simulink model "CBF_Attitude_with_feedback"  (R2020b)
settings: Solver=ode113  StartTime=0.0  StopTime=4  RelTol=1e-3
settings Model: Creator=kt012  LastModifiedBy=kt012

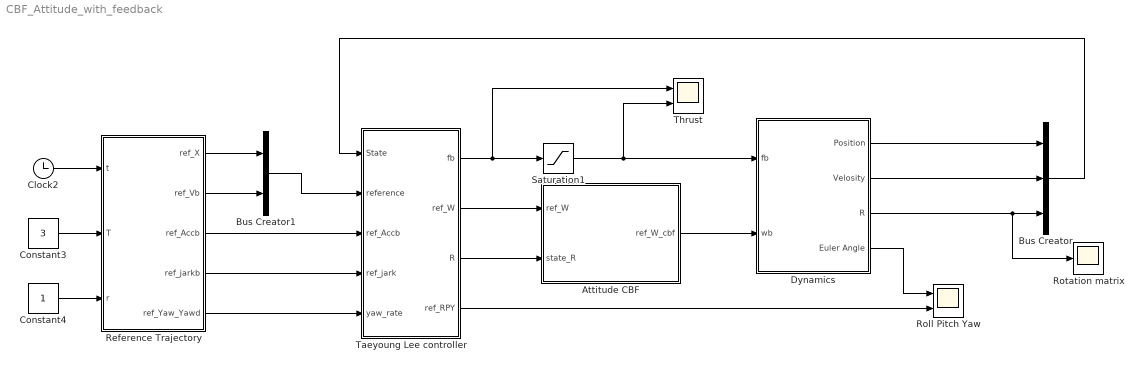
== system CBF_Attitude_with_feedback ==
  Attitude CBF : Subsystem
  Bus Creator : BusCreator  Inputs=3
  Bus Creator1 : BusCreator  Inputs=2
  Clock2 : Clock
  Constant3 : Constant  Value=3
  Constant4 : Constant
  Dynamics : Subsystem
  Reference Trajectory : MATLAB Function  TreatAsAtomicUnit=on
  Roll Pitch Yaw : Scope  NumInputPorts=2
  Rotation matrix : Scope
  Saturation1 : Saturate  UpperLimit=9.8*1.5
  Taeyoung Lee controller : Subsystem
  Thrust : Scope  NumInputPorts=2
  wires:
  Dynamics/2(Velosity) -> Bus Creator/2
  Taeyoung Lee controller/1(fb) -> Saturation1/1, Thrust/1
  Constant3/1 -> Reference Trajectory/2(T)
  Constant4/1 -> Reference Trajectory/3(r)
  Dynamics/4(Euler Angle) -> Roll Pitch Yaw/1
  Taeyoung Lee controller/2(ref_W) -> Attitude CBF/1(ref_W)
  Reference Trajectory/4(ref_jarkb) -> Taeyoung Lee controller/4(ref_jark)
  Reference Trajectory/1(ref_X) -> Bus Creator1/1
  Bus Creator/1 -> Taeyoung Lee controller/1(State)
  Reference Trajectory/2(ref_Vb) -> Bus Creator1/2
  Reference Trajectory/5(ref_Yaw_Yawd) -> Taeyoung Lee controller/5(yaw_rate)
  Dynamics/3(R) -> Rotation matrix/1, Bus Creator/3
  Reference Trajectory/3(ref_Accb) -> Taeyoung Lee controller/3(ref_Accb)
  Saturation1/1 -> Thrust/2, Dynamics/1(fb)
  Clock2/1 -> Reference Trajectory/1(t)
  Dynamics/1(Position) -> Bus Creator/1
  Bus Creator1/1 -> Taeyoung Lee controller/2(reference)
  Taeyoung Lee controller/4(ref_RPY) -> Roll Pitch Yaw/2
  Attitude CBF/1(ref_W_cbf) -> Dynamics/2(wb)
  Taeyoung Lee controller/3(R) -> Attitude CBF/2(state_R)

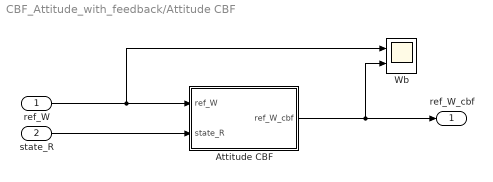
== system CBF_Attitude_with_feedback/Attitude CBF ==
  ref_W : Inport
  state_R : Inport  Port=2
  Attitude CBF : MATLAB Function  TreatAsAtomicUnit=on
  Wb : Scope  NumInputPorts=2
  ref_W_cbf : Outport
  wires:
  state_R/1 -> Attitude CBF/2(state_R)
  ref_W/1 -> Attitude CBF/1(ref_W), Wb/1
  Attitude CBF/1(ref_W_cbf) -> ref_W_cbf/1, Wb/2

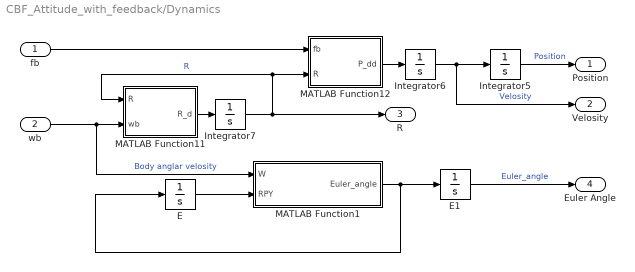
== system CBF_Attitude_with_feedback/Dynamics ==
  fb : Inport
  wb : Inport  Port=2
  E : Integrator  InitialCondition=[0 0 0];
  E1 : Integrator  InitialCondition=[0 0 0];
  Integrator5 : Integrator  InitialCondition=[0;0;0]
  Integrator6 : Integrator  InitialCondition=[0;0;0]
  Integrator7 : Integrator  InitialCondition=[1 0 0; 0 1 0; 0 0 1]
  MATLAB Function1 : MATLAB Function  TreatAsAtomicUnit=on
  MATLAB Function11 : MATLAB Function  TreatAsAtomicUnit=on
  MATLAB Function12 : MATLAB Function  TreatAsAtomicUnit=on
  Position : Outport
  Velosity : Outport  Port=2
  R : Outport  Port=3
  Euler Angle : Outport  Port=4
  wires:
  Integrator7/1 -> R/1, MATLAB Function12/2(R), MATLAB Function11/1(R)  "R"
  MATLAB Function11/1(R_d) -> Integrator7/1
  Integrator6/1 -> Velosity/1, Integrator5/1  "Velosity"
  MATLAB Function12/1(P_dd) -> Integrator6/1
  fb/1 -> MATLAB Function12/1(fb)
  Integrator5/1 -> Position/1  "Position"
  E/1 -> MATLAB Function1/2(RPY)
  E1/1 -> Euler Angle/1  "Euler_angle"
  MATLAB Function1/1(Euler_angle) -> E/1, E1/1
  wb/1 -> MATLAB Function1/1(W), MATLAB Function11/2(wb)  "Body anglar velosity"

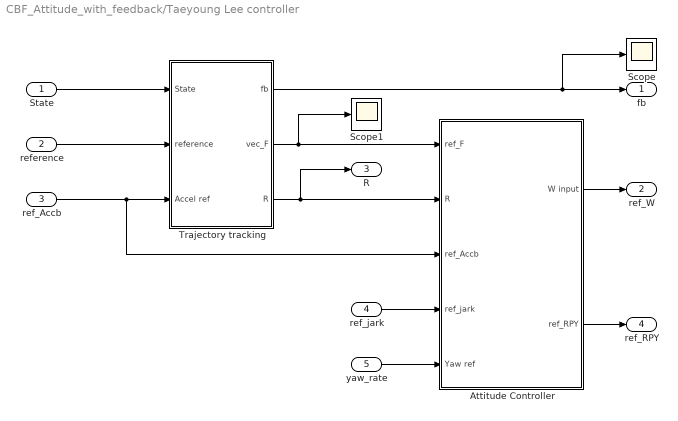
== system CBF_Attitude_with_feedback/Taeyoung Lee controller ==
  State : Inport
  reference : Inport  Port=2
  ref_Accb : Inport  Port=3
  ref_jark : Inport  Port=4
  yaw_rate : Inport  Port=5
  Attitude Controller : Subsystem
  Scope : Scope
  Scope1 : Scope
  Trajectory tracking : Subsystem
  fb : Outport
  ref_W : Outport  Port=2
  R : Outport  Port=3
  ref_RPY : Outport  Port=4
  wires:
  ref_Accb/1 -> Attitude Controller/3(ref_Accb), Trajectory tracking/3(Accel ref)
  ref_jark/1 -> Attitude Controller/4(ref_jark)
  reference/1 -> Trajectory tracking/2(reference)
  State/1 -> Trajectory tracking/1(State)
  yaw_rate/1 -> Attitude Controller/5(Yaw ref)
  Trajectory tracking/1(fb) -> Scope/1, fb/1
  Attitude Controller/1(W input) -> ref_W/1
  Trajectory tracking/2(vec_F) -> Scope1/1, Attitude Controller/1(ref_F)
  Attitude Controller/2(ref_RPY) -> ref_RPY/1
  Trajectory tracking/3(R) -> R/1, Attitude Controller/2(R)

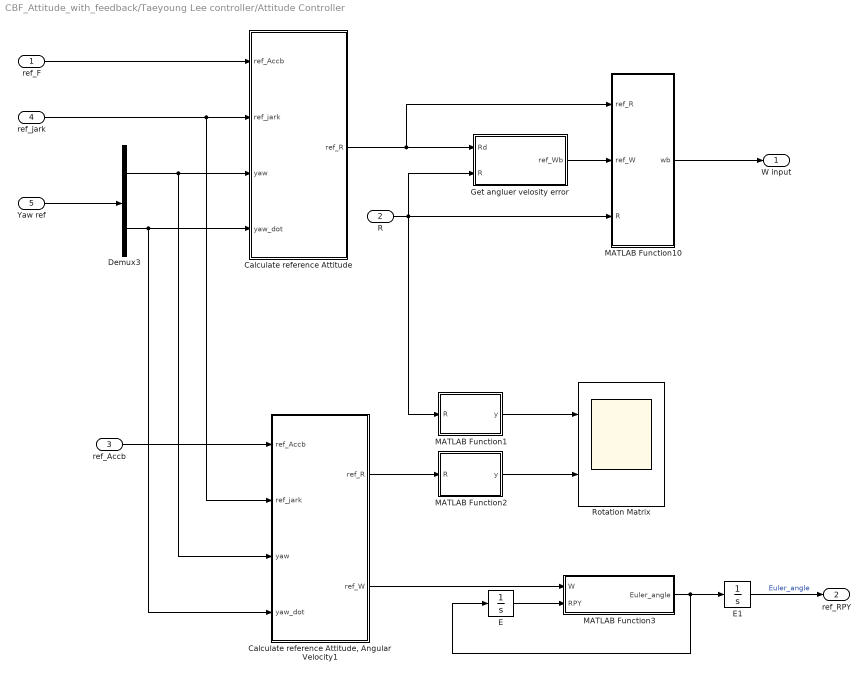
== system CBF_Attitude_with_feedback/Taeyoung Lee controller/Attitude Controller ==
  ref_F : Inport
  R : Inport  Port=2
  ref_Accb : Inport  Port=3
  ref_jark : Inport  Port=4
  Yaw ref : Inport  Port=5
  Calculate reference Attitude : MATLAB Function  TreatAsAtomicUnit=on
  "Calculate reference Attitude, Angular Velocity1" : MATLAB Function  TreatAsAtomicUnit=on
  Demux3 : Demux  Outputs=2
  E : Integrator  InitialCondition=[0 0 0];
  E1 : Integrator  InitialCondition=[0 0 0];
  Get angluer velosity error : Subsystem
  MATLAB Function1 : MATLAB Function  TreatAsAtomicUnit=on
  MATLAB Function10 : MATLAB Function  TreatAsAtomicUnit=on
  MATLAB Function2 : MATLAB Function  TreatAsAtomicUnit=on
  MATLAB Function3 : MATLAB Function  TreatAsAtomicUnit=on
  Rotation Matrix : Scope  NumInputPorts=2
  W input : Outport
  ref_RPY : Outport  Port=2
  wires:
  Demux3/2 -> Calculate reference Attitude/4(yaw_dot), "Calculate reference Attitude, Angular Velocity1"/4(yaw_dot)
  Yaw ref/1 -> Demux3/1
  Demux3/1 -> Calculate reference Attitude/3(yaw), "Calculate reference Attitude, Angular Velocity1"/3(yaw)
  ref_F/1 -> Calculate reference Attitude/1(ref_Accb)
  ref_jark/1 -> Calculate reference Attitude/2(ref_jark), "Calculate reference Attitude, Angular Velocity1"/2(ref_jark)
  MATLAB Function10/1(wb) -> W input/1
  MATLAB Function1/1(y) -> Rotation Matrix/1
  MATLAB Function2/1(y) -> Rotation Matrix/2
  ref_Accb/1 -> "Calculate reference Attitude, Angular Velocity1"/1(ref_Accb)
  "Calculate reference Attitude, Angular Velocity1"/1(ref_R) -> MATLAB Function2/1(R)
  "Calculate reference Attitude, Angular Velocity1"/2(ref_W) -> MATLAB Function3/1(W)
  MATLAB Function3/1(Euler_angle) -> E/1, E1/1
  E/1 -> MATLAB Function3/2(RPY)
  E1/1 -> ref_RPY/1  "Euler_angle"
  Calculate reference Attitude/1(ref_R) -> MATLAB Function10/1(ref_R), Get angluer velosity error/1(Rd)
  R/1 -> Get angluer velosity error/2(R), MATLAB Function10/3(R), MATLAB Function1/1(R)
  Get angluer velosity error/1(ref_Wb) -> MATLAB Function10/2(ref_W)

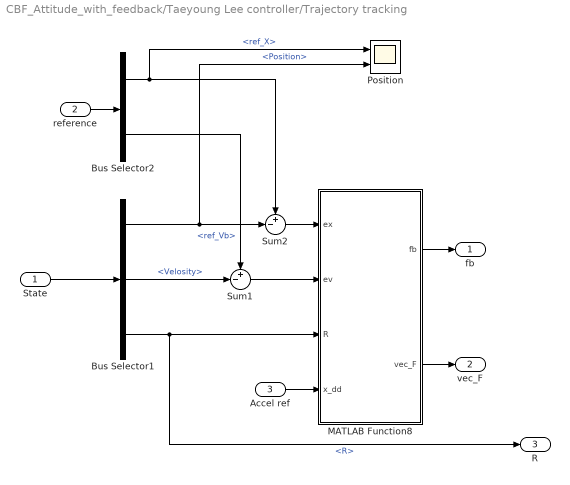
== system CBF_Attitude_with_feedback/Taeyoung Lee controller/Trajectory tracking ==
  State : Inport
  reference : Inport  Port=2
  Accel ref : Inport  Port=3
  Bus Selector1 : BusSelector  OutputSignals=Position,Velosity,R
  Bus Selector2 : BusSelector  OutputSignals=ref_X,ref_Vb
  MATLAB Function8 : MATLAB Function
  Position : Scope  NumInputPorts=2
  Sum1 : Sum  Inputs=+-|
  Sum2 : Sum  Inputs=+-|
  fb : Outport
  vec_F : Outport  Port=2
  R : Outport  Port=3
  wires:
  State/1 -> Bus Selector1/1
  Accel ref/1 -> MATLAB Function8/4(x_dd)
  reference/1 -> Bus Selector2/1
  MATLAB Function8/1(fb) -> fb/1
  MATLAB Function8/2(vec_F) -> vec_F/1
  Bus Selector2/2 -> Sum1/1  "<ref_Vb>"
  Bus Selector1/2 -> Sum1/2  "<Velosity>"
  Bus Selector2/1 -> Position/1, Sum2/1  "<ref_X>"
  Bus Selector1/1 -> Position/2, Sum2/2  "<Position>"
  Sum2/1 -> MATLAB Function8/1(ex)
  Bus Selector1/3 -> R/1, MATLAB Function8/3(R)  "<R>"
  Sum1/1 -> MATLAB Function8/2(ev)

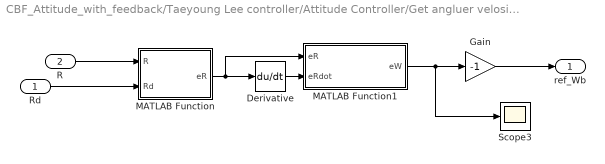
== system CBF_Attitude_with_feedback/Taeyoung Lee controller/Attitude Controller/Get angluer velosity error ==
  Rd : Inport
  R : Inport  Port=2
  Derivative : Derivative
  Gain : Gain  Gain=-1
  MATLAB Function : MATLAB Function  TreatAsAtomicUnit=on
  MATLAB Function1 : MATLAB Function  TreatAsAtomicUnit=on
  Scope3 : Scope
  ref_Wb : Outport
  wires:
  R/1 -> MATLAB Function/1(R)
  MATLAB Function/1(eR) -> MATLAB Function1/1(eR), Derivative/1
  MATLAB Function1/1(eW) -> Scope3/1, Gain/1
  Gain/1 -> ref_Wb/1
  Derivative/1 -> MATLAB Function1/2(eRdot)
  Rd/1 -> MATLAB Function/2(Rd)

== matlab function CBF_Attitude_with_feedback/Taeyoung Lee controller/Trajectory tracking/MATLAB Function8 ==
  data: ex input; fb output; ev input; R input; x_dd input; vec_F output
function [fb, vec_F]= fcn(ex,ev,R, x_dd)
ev_d = [0 0 0]';
ex_d = [0 0 0]';
fb = 0;
vec_F = [0 0 0]';
m = 1.0;
e3 = [0;0;1];

kx_x = 10;
kx_y = 10;
kx_z = 10;

kv_x = 10;
kv_y = 10;
kv_z = 10;

ex_x = kx_x*ex(1);
ex_y = kx_y*ex(2);
ex_z = kx_z*ex(3);
ex_d = [ex_x; ex_y; ex_z];

ev_x = kv_x*ev(1);
ev_y = kv_y*ev(2);
ev_z = kv_z*ev(3);
ev_d = [ev_x; ev_y; ev_z];
fb = dot(ex_d + ev_d + m*x_dd, R*e3);
tmp = ex_d + ev_d + m*x_dd;
if tmp(3) <= 0.0001
    tmp(3) = 0.0001;
end
vec_F = tmp;

== matlab function CBF_Attitude_with_feedback/Taeyoung Lee controller/Attitude Controller/MATLAB Function10 ==
  data: ref_R input; ref_W input; R input; wb output
function wb = fcn(ref_R,ref_W, R)
R_T = R';
Rd_T = ref_R';
eR = (Rd_T*R - R_T*ref_R)/2;

kR = 20;
wx = ref_W(1);
wy = ref_W(2);
wz = ref_W(3);
wd = [0 -wz wy; 
      wz 0 -wx;
      -wy wx 0];
u = -kR * eR + wd;

wb = u;

== matlab function CBF_Attitude_with_feedback/Dynamics/MATLAB Function12 ==
  data: fb input; P_dd output; R input
function P_dd = fcn(fb,R)
e3 = [0;0;1];
g = 9.8;
m = 1;

u = (fb*R*e3/m) - g*e3 ;

P_dd = u;

== matlab function CBF_Attitude_with_feedback/Reference Trajectory ==
  data: ref_X output; ref_Vb output; ref_Accb output; ref_jarkb output; t input; ref_Yaw_Yawd output; T input; r input
  function [ref_X, ref_Vb, ref_Accb, ref_jarkb, ref_Yaw_Yawd] = fcn(t,T,r)
% 軌道生成
w = 2 * pi/T;     
% 軌道生成（直線移動）
ref_X = [r*sin(w*t);0; 0];
ref_Vb = [r*w*cos(w*t); 0; 0];
ref_Accb = [-r*w^2*sin(w*t); 0; 9.8];
ref_jarkb = [-r*w^3*cos(w*t);0;0];
ref_Yaw_Yawd = [0, 0]'; 

% % 軌道生成（直線移動）
% ref_X = [r/(1+exp(-t));0; 0];
% ref_Vb = [(1-ref_X(1))*ref_X(1); 0; 0];
% ref_Accb = [(1-ref_Vb(1))*ref_Vb(1); 0; 9.8];
% ref_jarkb = [(1-ref_Accb(1))*ref_Accb(1);0;0];
% ref_Yaw_Yawd = [0, 0]';
% % 軌道生成
w = 2 * pi/T;     
% % 軌道生成（直線移動）
% ref_X = [1;0; 0];
% ref_Vb = [0; 0; 0];
% ref_Accb = [0; 0; 9.8];
% ref_jarkb = [-r*w^3*cos(w*t);0;0];
% ref_Yaw_Yawd = [0, 0]'; 

% 軌道生成（直線移動）
% ref_X = [4*t^2;0; 0];
% ref_Vb = [8*t; 0; 0];
% ref_Accb = [8; 0; 9.8];
% ref_jarkb = [0;0;0];
% ref_Yaw_Yawd = [0, 0]';

== matlab function CBF_Attitude_with_feedback/Taeyoung Lee controller/Attitude Controller/Calculate reference Attitude ==
  data: ref_R output; ref_Accb input; ref_jark input; yaw input; yaw_dot input
function ref_R= fcn(ref_Accb, ref_jark, yaw, yaw_dot)

% Flat Outputから内部状態と入力揚力を計算


Xc = [cos(yaw) sin(yaw) 0]';          % よー角のベクトル　Rc(3)
Yc = [-sin(yaw) cos(yaw) 0]';
dXc = yaw_dot * Yc; % よー角のベクトルの微分
dYc = -yaw_dot * Xc; 

% 所望の姿勢を計算している
% 軌道の加速度のベクトル: b3 を計算
Zb = ref_Accb / norm(ref_Accb);    
%
Yb = cross(Zb, Xc)/norm(cross(Zb, Xc));
Xb = cross(Yb, Zb);
% Xb = cross(Yc, Zb)/norm(cross(Yc, Zb));
% Yb = cross(Zb, Xb);
ref_R = [Xb Yb Zb] ;




% % 加加速度ベクトルを計算
% dfZb = ref_jark;
%   
% % 目標の姿勢のz軸方向のベクトルの微分を計算
% dZb = dfZb/norm(ref_Accb) - ref_Accb * dot(ref_Accb, dfZb)/norm(ref_Accb)^3; % Zb_dot---------- dot(　fb1/norm(fb1) )
% 
% % 目標の姿勢のx軸方向のベクトルを計算
% dnorm_Zb_Xc2 = norm(cross(dYc, Zb) + cross(Yc, dZb));
% dXb = (cross(dYc, Zb) + cross(Yc, dZb))/dnorm_Zb_Xc2 - cross(Yc, Zb) * dot(cross(Yc, Zb),( cross(dYc, Zb) + cross(Yc, dZb)))/dnorm_Zb_Xc2^3;
%    
% % 目標の姿勢のy軸方向のベクトルを計算
% dYb = cross(dZb, Xb) + cross(Zb, dXb) ;  %dot_b2 = dotb3とb1 の外積と　b3とdot_b1の外積　の和　--------- dot(cross(b3, b1))
% 
% 
% wy = dot(Xb, ref_jark) / dot(Zb, ref_Accb);
% wx = - dot(Yb, ref_jark) / dot(Zb, ref_Accb);
% wz = (yaw_dot * dot(Xc, Xb) + wy * dot(Yc, Zb))/norm(cross(Yc, Zb));
% ref_W = [wx wy wz];

== matlab function CBF_Attitude_with_feedback/Attitude CBF/Attitude CBF ==
  data: ref_W input; state_R input; ref_W_cbf output
function ref_W_cbf = fcn(ref_W, state_R)
ref_W = [ref_W(3, 2), -ref_W(3, 1), ref_W(2, 1)]';
theta = 0.5;
coder.extrinsic('quadprog')
tmp = zeros(3, 1);
e3 = [0; 0; 1];
e3_wedge = [0 -1 0; 1 0 0; 0 0 0];
H = eye(3);
f = -ref_W;
% ref_W
A = e3'*state_R*e3_wedge;
B = 10*(e3'*state_R*e3 - cos(theta));

tmp  = quadprog(H, f, A, B);
ref_W_cbf = [0      -tmp(3)   tmp(2); 
             tmp(3)  0       -tmp(1); 
             -tmp(2) tmp(1)   0]
A*tmp
B
end

== matlab function CBF_Attitude_with_feedback/Dynamics/MATLAB Function11 ==
  data: R input; wb input; R_d output
function R_d = fcn(R,wb)
u = R * wb;
R_d = u;

== matlab function CBF_Attitude_with_feedback/Taeyoung Lee controller/Attitude Controller/MATLAB Function2 ==
  data: R input; y output
function y = fcn(R)
Rtranspose = R';
eR = (R - Rtranspose)/2;

y = [eR(3, 2) -eR(3, 1) eR(2, 1)]';

== matlab function CBF_Attitude_with_feedback/Taeyoung Lee controller/Attitude Controller/MATLAB Function1 ==
  data: R input; y output
function y = fcn(R)
Rtranspose = R';
eR = (R - Rtranspose)/2;

y = [eR(3, 2) -eR(3, 1) eR(2, 1)]';

== matlab function CBF_Attitude_with_feedback/Taeyoung Lee controller/Attitude Controller/Calculate reference Attitude, Angular Velocity1 ==
  data: ref_R output; ref_W output; ref_Accb input; ref_jark input; yaw input; yaw_dot input
function [ref_R,ref_W]= fcn(ref_Accb, ref_jark, yaw, yaw_dot)

% Flat Outputから内部状態と入力揚力を計算


Xc = [cos(yaw) sin(yaw) 0]';          % よー角のベクトル　Rc(3)
Yc = [-sin(yaw) cos(yaw) 0]';
dXc = yaw_dot * Yc; % よー角のベクトルの微分
dYc = -yaw_dot * Xc; 

% 所望の姿勢を計算している
% 軌道の加速度のベクトル: b3 を計算
Zb = ref_Accb / norm(ref_Accb);   
%
Yb = cross(Zb, Xc)/norm(cross(Zb, Xc));
Xb = cross(Yb, Zb);
% Xb = cross(Yc, Zb)/norm(cross(Yc, Zb));
% Yb = cross(Zb, Xb);
ref_R = [Xb Yb Zb] ;
% 加加速度ベクトルを計算
dfZb = ref_jark;
  
% 目標の姿勢のz軸方向のベクトルの微分を計算
dZb = dfZb/norm(ref_Accb) - ref_Accb * dot(ref_Accb, dfZb)/norm(ref_Accb)^3; % Zb_dot---------- dot(　fb1/norm(fb1) )

% 目標の姿勢のx軸方向のベクトルを計算
dnorm_Zb_Xc2 = norm(cross(dYc, Zb) + cross(Yc, dZb));
dXb = (cross(dYc, Zb) + cross(Yc, dZb))/dnorm_Zb_Xc2 - cross(Yc, Zb) * dot(cross(Yc, Zb),( cross(dYc, Zb) + cross(Yc, dZb)))/dnorm_Zb_Xc2^3;
   
% 目標の姿勢のy軸方向のベクトルを計算
dYb = cross(dZb, Xb) + cross(Zb, dXb) ;  %dot_b2 = dotb3とb1 の外積と　b3とdot_b1の外積　の和　--------- dot(cross(b3, b1))


wy = dot(Xb, ref_jark) / dot(Zb, ref_Accb);
wx = - dot(Yb, ref_jark) / dot(Zb, ref_Accb);
wz = (yaw_dot * dot(Xc, Xb) + wy * dot(Yc, Zb))/norm(cross(Yc, Zb));
ref_W = [wx wy wz];

== matlab function CBF_Attitude_with_feedback/Taeyoung Lee controller/Attitude Controller/MATLAB Function3 ==
  data: W input; Euler_angle output; RPY input
function Euler_angle = fcn(W, RPY)
roll = RPY(1);
pitch = RPY(2);
yaw = RPY(3);
rollS = sin(roll); rollC = cos(roll);           
pitchS = sin(pitch); pitchC = cos(pitch);       


Euler_angle = pinv([1 0 -pitchS;
     0 rollC  pitchC * rollS;
     0 -rollS pitchC * rollC]) * W';

== matlab function CBF_Attitude_with_feedback/Dynamics/MATLAB Function1 ==
  data: W input; Euler_angle output; RPY input
function Euler_angle = fcn(W, RPY)
W = [W(3, 2), -W(3, 1), W(2, 1)]';
roll = RPY(1);
pitch = RPY(2);
yaw = RPY(3);
rollS = sin(roll); rollC = cos(roll);           
pitchS = sin(pitch); pitchC = cos(pitch);       


Euler_angle = pinv([1 0 -pitchS;
     0 rollC  pitchC * rollS;
     0 -rollS pitchC * rollC]) * W;

== matlab function CBF_Attitude_with_feedback/Taeyoung Lee controller/Attitude Controller/Get angluer velosity error/MATLAB Function ==
  data: R input; eR output; Rd input
function eR = fcn(R, Rd)
R = eye(3);
eR = Rd'*R;

== matlab function CBF_Attitude_with_feedback/Taeyoung Lee controller/Attitude Controller/Get angluer velosity error/MATLAB Function1 ==
  data: eR input; eW output; eRdot input
function eW = fcn(eR, eRdot)

tmp= pinv(eR) * eRdot;
eW = [tmp(3, 2) tmp(1, 3) tmp(2, 1)]';
